simulink subsystem "Find_Catmull_Rom_Pos"  (R2023b)
settings: Solver=VariableStepAuto  StartTime=0.0  StopTime=10.0  RelTol=1e-3
settings Model: Creator=FIRSTMentor  LastModifiedBy=ander

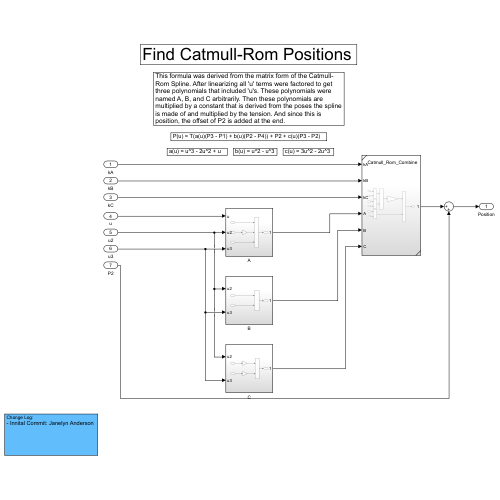
[thumbnail: Simulink's stored preview of the top-level diagram]
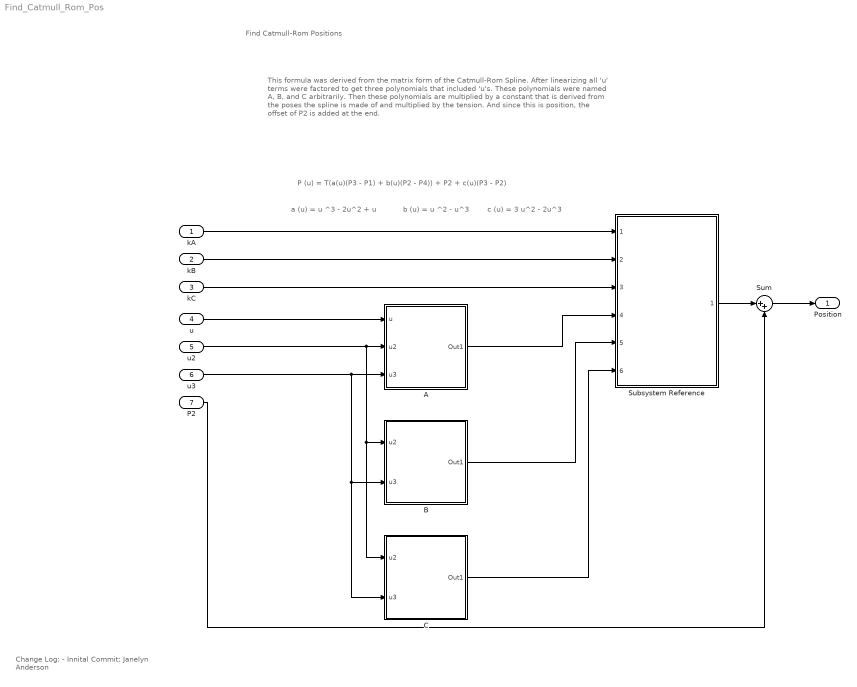
== system Find_Catmull_Rom_Pos ==
  note: Change Log:
      | - Innital Commit: Janelyn Anderson
  note: Find Catmull-Rom Positions
  note: P (u) = T(a(u)(P3 - P1) + b(u)(P2 - P4)) + P2 + c(u)(P3 - P2)
  note: This formula was derived from the matrix form of the Catmull-Rom Spline. After linearizing all 'u' terms were factored to get three polynomials that included 'u's. These polynomials were named A, B, and C arbitrarily. Then these polynomials are multiplied by a constant that is derived from the poses the spline is made of and multiplied by the tension. And since this is position, the offset of P2 is added at the end.
  note: c (u) = 3 u^2 - 2u^3
  note: b (u) = u ^2 - u^3
  note: a (u) = u ^3 - 2u^2 + u
  kA : Inport  PortDimensions=[1 2]
  kB : Inport  Port=2  PortDimensions=[1 2]
  kC : Inport  Port=3  PortDimensions=[1 2]
  u : Inport  Port=4  PortDimensions=1
  u2 : Inport  Port=5  PortDimensions=1
  u3 : Inport  Port=6  PortDimensions=1
  P2 : Inport  Port=7  PortDimensions=[1 2]
  A : Subsystem
  B : Subsystem
  C : Subsystem
  Subsystem Reference : Subsystem  ReferencedSubsystem=Catmull_Rom_Combine
  Sum : Sum  Inputs=|++
  Position : Outport
  wires:
  Subsystem Reference/1 -> Sum/1
  A/1(Out1) -> Subsystem Reference/4
  kB/1 -> Subsystem Reference/2
  Sum/1 -> Position/1
  kA/1 -> Subsystem Reference/1
  C/1(Out1) -> Subsystem Reference/6
  P2/1 -> Sum/2
  B/1(Out1) -> Subsystem Reference/5
  kC/1 -> Subsystem Reference/3
  u3/1 -> C/2(u3), B/2(u3), A/3(u3)
  u/1 -> A/1(u)
  u2/1 -> C/1(u2), B/1(u2), A/2(u2)

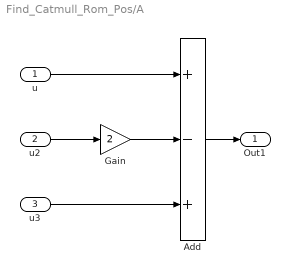
== system Find_Catmull_Rom_Pos/A ==
  u : Inport
  u2 : Inport  Port=2
  u3 : Inport  Port=3
  Add : Sum  Inputs=+-+
  Gain : Gain  Gain=2
  Out1 : Outport
  wires:
  u3/1 -> Add/3
  Gain/1 -> Add/2
  u2/1 -> Gain/1
  u/1 -> Add/1
  Add/1 -> Out1/1

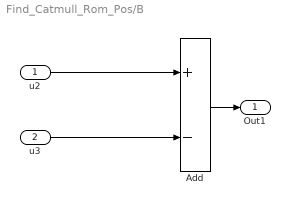
== system Find_Catmull_Rom_Pos/B ==
  u2 : Inport
  u3 : Inport  Port=2
  Add : Sum  Inputs=+-
  Out1 : Outport
  wires:
  u2/1 -> Add/1
  u3/1 -> Add/2
  Add/1 -> Out1/1

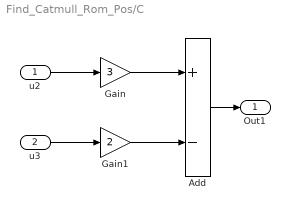
== system Find_Catmull_Rom_Pos/C ==
  u2 : Inport
  u3 : Inport  Port=2
  Add : Sum  Inputs=+-
  Gain : Gain  Gain=3
  Gain1 : Gain  Gain=2
  Out1 : Outport
  wires:
  Add/1 -> Out1/1
  Gain1/1 -> Add/2
  Gain/1 -> Add/1
  u3/1 -> Gain1/1
  u2/1 -> Gain/1
